simulink model "simpleTVCRocketModel"  (R2021b)
settings: Solver=VariableStepAuto  StartTime=0.0  StopTime=10  RelTol=1e-3
PostLoadFcn:
  | VSS_MODE = 0;
model workspace (MAT data in the model file):
  op_trim6 = opcond.OperatingReport
  op_trim6.Outputs_ = opcond.OutputReport
  op_trim6.Outputs_.yspec_ = 0
  op_trim6.Outputs_.Block_ = 'simpleTVCRocketModel/Theta'
  op_trim6.Outputs_.PortWidth_ = 1
  op_trim6.Outputs_.PortNumber_ = NaN
  op_trim6.Outputs_.Known_ = 0
  op_trim6.Outputs_.Min_ = -Inf
  op_trim6.Outputs_.Max_ = Inf
  op_trim6.TerminationString_ = 'Operating point specifications were successfully met.'
  op_trim6.OptimizationOutput_.iterations = 1
  op_trim6.OptimizationOutput_.funcCount = 9
  op_trim6.OptimizationOutput_.lssteplength = 1
  op_trim6.OptimizationOutput_.stepsize = 0
  op_trim6.OptimizationOutput_.algorithm = 'active-set'
  op_trim6.OptimizationOutput_.firstorderopt = 0
  op_trim6.OptimizationOutput_.constrviolation = 0
  op_trim6.OptimizationOutput_.message = '
    | Local minimum found that satisfies the constraints.
    | 
    | Optimization completed because the objective function is non-decreasing in 
    | feasible directions, to within the value of the optimality tolerance,
    | and constraints are satisfied to within the  value of the constraint tolerance.
    | 
    | <stopping criteria details>
    | 
    | Optimization completed: The first-order optimality measure, 0.000000e+00, is less
    | than options.OptimalityTolerance = 1.000000e-06, and the maximum constraint violation,
    | 0.000000e+00,is less than options.ConstraintTolerance = 1.000000e-06.
    | 
    | '
  op_trim6.OptimizationOutput_.bestfeasible.x = [0; 0; 0; 0; 0; 0; 0; 0]
  op_trim6.OptimizationOutput_.bestfeasible.fval = 0
  op_trim6.OptimizationOutput_.bestfeasible.constrviolation = 0
  op_trim6.OptimizationOutput_.bestfeasible.firstorderopt = 0
  op_trim6.OptimizationOutput_.progress = {'<font face="monospaced"; size=3>', 'Optimizing to solve for all desired dx/dt=0, x(k+1)-x(k)=0, and y=ydes.', ' ', '(Maximum Error)  Block', ' ---------------------------------------------------------', '(0.00000e+00) There are no errors in the operating point search constraints.', '(0.00000e+00) There are no errors in the operating point search constraints.', ' ', 'Operating point specifications were successfully met.'}
  op_trim6.Model_ = 'simpleTVCRocketModel'
  op_trim6.States_(1) = opcond.StateReport
  op_trim6.States_(1).dx_ = [0; 0]
  op_trim6.States_(1).Nx_ = 2
  op_trim6.States_(1).Block_ = 'simpleTVCRocketModel/RocketModel/ASB Rocket Model/Rocket Model/Position'
  op_trim6.States_(1).x_ = [0; 0]
  op_trim6.States_(1).SteadyState_ = [0; 0]
  op_trim6.States_(1).dxMin_ = [-Inf; -Inf]
  op_trim6.States_(1).dxMax_ = [Inf; Inf]
  op_trim6.States_(1).Known_ = [0; 0]
  op_trim6.States_(1).Min_ = [-Inf; -Inf]
  op_trim6.States_(1).Max_ = [Inf; Inf]
  op_trim6.States_(2) = opcond.StateReport
  op_trim6.States_(2).Nx_ = 1
  op_trim6.States_(2).Block_ = 'simpleTVCRocketModel/RocketModel/ASB Rocket Model/Rocket Model/Theta'
  op_trim6.States_(2).SteadyState_ = 1
  op_trim6.States_(2).dxMin_ = -Inf
  op_trim6.States_(2).dxMax_ = Inf
  op_trim6.States_(2).Known_ = 1
  op_trim6.States_(2).Min_ = -Inf
  op_trim6.States_(2).Max_ = Inf
  op_trim6.States_(3) = opcond.StateReport
  op_trim6.States_(3).dx_ = [0; -6.85666666667]
  op_trim6.States_(3).Nx_ = 2
  op_trim6.States_(3).Block_ = 'simpleTVCRocketModel/RocketModel/ASB Rocket Model/Rocket Model/U,w'
  op_trim6.States_(3).x_ = [0; 0]
  op_trim6.States_(3).SteadyState_ = [0; 0]
  op_trim6.States_(3).dxMin_ = [-Inf; -Inf]
  op_trim6.States_(3).dxMax_ = [Inf; Inf]
  op_trim6.States_(3).Known_ = [0; 0]
  op_trim6.States_(3).Min_ = [-Inf; -Inf]
  op_trim6.States_(3).Max_ = [Inf; Inf]
  op_trim6.States_(4) = opcond.StateReport
  op_trim6.States_(4).dx_ = 0
  op_trim6.States_(4).Nx_ = 1
  op_trim6.States_(4).Block_ = 'simpleTVCRocketModel/RocketModel/ASB Rocket Model/Rocket Model/q'
  op_trim6.States_(4).SteadyState_ = 0
  op_trim6.States_(4).dxMin_ = -Inf
  op_trim6.States_(4).dxMax_ = Inf
  op_trim6.States_(4).Known_ = 0
  op_trim6.States_(4).Min_ = -Inf
  op_trim6.States_(4).Max_ = Inf
  op_trim6.States_(5) = opcond.StateReport
  op_trim6.States_(5).Nx_ = 1
  op_trim6.States_(5).Block_ = 'simpleTVCRocketModel/Controller/PID Controller/Filter/Cont. Filter/Filter'
  op_trim6.States_(5).SteadyState_ = 0
  op_trim6.States_(5).dxMin_ = -Inf
  op_trim6.States_(5).dxMax_ = Inf
  op_trim6.States_(5).Known_ = 0
  op_trim6.States_(5).Min_ = -Inf
  op_trim6.States_(5).Max_ = Inf
  op_trim6.States_(6) = opcond.StateReport
  op_trim6.States_(6).Nx_ = 1
  op_trim6.States_(6).Block_ = 'simpleTVCRocketModel/Controller/PID Controller/Integrator/Continuous/Integrator'
  op_trim6.States_(6).SteadyState_ = 0
  op_trim6.States_(6).dxMin_ = -Inf
  op_trim6.States_(6).dxMax_ = Inf
  op_trim6.States_(6).Known_ = 0
  op_trim6.States_(6).Min_ = -Inf
  op_trim6.States_(6).Max_ = Inf
  op_trim6.Inputs_ = opcond.InputReport
  op_trim6.Inputs_.Block_ = 'simpleTVCRocketModel/u'
  op_trim6.Inputs_.PortWidth_ = 1
  op_trim6.Inputs_.PortDimensions_ = [1 1]
  op_trim6.Inputs_.Known_ = 0
  op_trim6.Inputs_.Min_ = -Inf
  op_trim6.Inputs_.Max_ = Inf
libraries: simulink_extras x2, aerolibadyn x1, aerolibconvert2 x1, aerolibanim x1, slpidlib x1, shared3dof x1, simulink x1
settings Model: Creator=joebarnard  LastModifiedBy=willi
settings SolverCC: AlgebraicLoopSolver=TrustRegion
settings DataIOCC: ExternalInput=getinputstruct(op_trim6)  InitialState=getstatestruct(op_trim6)  LoadExternalInput=on  LoadInitialState=on
settings DebuggingCC: SFMachineParentedDataDiag=warning
settings ExplorerConfigSet: InternalSimMechanicsExplorerSettings="<ExplorerConfiguration><canonicalview>default</canonicalview><AnimationSetting><BasePlaybackSpeed>1.0</BasePlaybackSpeed><PlaybackSpeedFactor>1.0</PlaybackSpeedFactor></AnimationSetting><TilePanel><TileInfo><Tiles Columns=\"2\" Count=\"3\" Rows=\"2\"><Column Weight=\"0.5\"/><Column Weight=\"0.5\"/><Row Weight=\"0.5164\"/><Row Weight=\"0.4836\"/><Tile Height=\"1\" Width=\"2\" X=\"0\" Y=\"0\"/><Tile Height=\"1\" Width=\"1\" X=\"0\" Y=\"1\"/><Tile Height=\"1\" Width=\"1\" X=\"1\" Y=\"1\"/></Tiles></TileInfo><SceneInfo><SceneViewer><BGColor><R>0.60000002384185791</R><G>0.60000002384185791</G><B>0.60000002384185791</B></BGColor><Camera><DoPerspective>on</DoPerspective><Position><X>0.0234785756067064089</X><Y>-5.49998084299828705</Y><Z>1.77140121776666781</Z></Position><Center><X>0.0234785756067064089</X><Y>-4.49998084299828705</Y><Z>1.77140121776666781</Z></Center><Up><X>0</X><Y>0</Y><Z>1</Z></Up><ViewLimDist>1</ViewLimDist><YLim>0.466307658154998583</YLim><XLim>1.57644492475456621</XLim></Camera></SceneViewer><SceneViewer><BGColor><R>0.60000002384185791</R><G>0.60000002384185791</G><B>0.60000002384185791</B></BGColor><Camera><DoPerspective>off</DoPerspective><Position><X>1.24658653086195947e-06</X><Y>70.9082318296519531</Y><Z>0.982810102945052222</Z></Position><Center><X>1.24658653086195947e-06</X><Y>-1.81285147970999816e-06</Y><Z>0.982810102945052222</Z></Center><Up><X>0</X><Y>0</Y><Z>1</Z></Up><ViewLimDist>1</ViewLimDist><YLim>28.7116613418530342</YLim><XLim>51.5</XLim></Camera></SceneViewer><SceneViewer><BGColor><R>0.60000002384185791</R><G>0.60000002384185791</G><B>0.60000002384185791</B></BGColor><Camera><DoPerspective>on</DoPerspective><Position><X>0</X><Y>0</Y><Z>3.5</Z></Position><Center><X>0</X><Y>-2.22044604925031308e-16</Y><Z>2.5</Z></Center><Up><X>1</X><Y>0</Y><Z>0</Z></Up><ViewLimDist>1</ViewLimDist><YLim>0.466307658154998583</YLim><XLim>0.836414309469997397</XLim></Camera></SceneViewer></SceneInfo></TilePanel><MechEditorPanel><Cameras><Camera><Id>Camera1</Id><Value><Name>trackCam</Name><NativeCamera><PositionTrackingFeature>RocketModel.Simscape_Rocket_Model.trackCam.R</PositionTrackingFeature><CenterTrackingFeature>RocketModel.Simscape_Rocket_Model.trackCam.R</CenterTrackingFeature><UpVectorTrackingFeature>RocketModel.Simscape_Rocket_Model.trackCam.R</UpVectorTrackingFeature><CenterTrackingOrigin>off</CenterTrackingOrigin><CenterTrackingDirection>-Y</CenterTrackingDirection><UpVectorTrackingDirection>+X</UpVectorTrackingDirection></NativeCamera></Value></Camera><Camera><Id>Camera2</Id><Value><Name>sideTrack</Name><NativeCamera><PositionTrackingFeature>RocketModel.Simscape_Rocket_Model.Camera1.R</PositionTrackingFeature><CenterTrackingFeature>RocketModel.Simscape_Rocket_Model.Camera1.R</CenterTrackingFeature><UpVectorTrackingFeature>RocketModel.Simscape_Rocket_Model.Camera1.R</UpVectorTrackingFeature><CenterTrackingOrigin>off</CenterTrackingOrigin><CenterTrackingDirection>+X</CenterTrackingDirection><UpVectorTrackingDirection>+Y</UpVectorTrackingDirection></NativeCamera></Value></Camera></Cameras><GfxPanelCameraMap><MapElement CameraMLId=\"Camera2\" GfxPanelIndex=\"0\"/><MapElement CameraMLId=\"Camera1\" GfxPanelIndex=\"2\"/></GfxPanelCameraMap><VideoCreator><PlaybackSpeedRatio>1.0</PlaybackSpeedRatio><FrameRate>30</FrameRate><VideoFormat>Motion JPEG AVI</VideoFormat><FrameSize>auto</FrameSize></VideoCreator></MechEditorPanel></ExplorerConfiguration>"

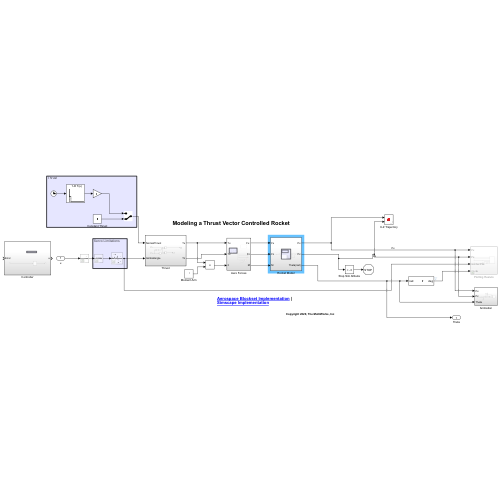
[thumbnail: Simulink's stored preview of the top-level diagram]
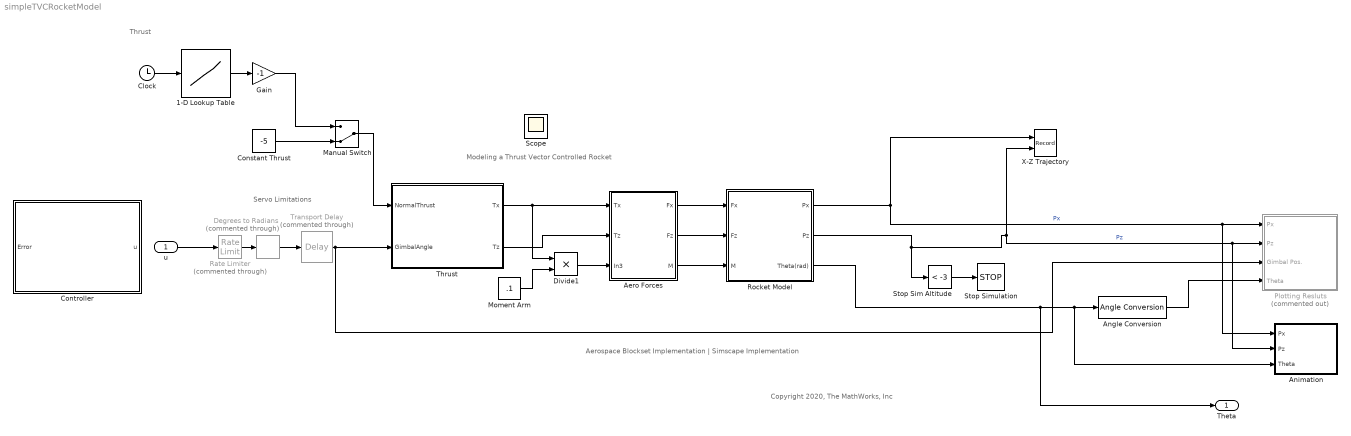
== system simpleTVCRocketModel ==
  note: Servo Limitations
  note: Thrust
  note: Aerospace Blockset Implementation | Simscape Implementation
  note: Modeling a Thrust Vector Controlled Rocket
  note: Copyright 2020, The MathWorks, Inc
  u : Inport
  1-D Lookup Table : Lookup_n-D  NumberOfTableDimensions=1  BreakpointsForDimension1=linspace(0,16.14, 539)  Table=|  InternalRulePriority=Speed  RndMeth=Simplest  InputSameDT=on
      | [0
      | 1.69832354141853
      | 2.47292485439563
      | 4.39373828780983
      | 6.77722955360763
      | 9.10300000000000
      | 11.3977773557748
      | 11.6140807786675
      | 8.98706894846169
      | 6.10838111022478
      | 5.33611774178522
      | 5.01684267037569
      | 5.12969642924522
      | 4.72506262341681
      | 4.73496687053046
      | 4.76034152927576
      | 4.77096696821312
      | 4.76949450279542
      | 4.76619751371507
      | 4.76157438946575
      | 4.75612351854116
      | 4.75034328943497
      | 4.74465776015659
      | 4.73771752958070
      | 4.72923958998768
      | 4.71974568770069
      | 4.70975756904293
      | 4.69979698033756
      | 4.69038566790776
      | 4.68204537807671
      | 4.67529785716758
      | 4.67027632477041
      | 4.66550157069833
      | 4.66080212375550
      | 4.65621865771085
      | 4.65179184633330
      | 4.64756236339179
      | 4.64357088265525
      | 4.63985807789262
      | 4.63646462287282
      | 4.63343119136480
      | 4.63079845713747
      | 4.62860709395979
      | 4.62689777560066
      | 4.62571117582904
      | 4.62508796841385
      | 4.62500000000000
      | 4.62500000000000
      | 4.62500000000000
      | 4.62500000000000
      | 4.62500000000000
      | 4.62500000000000
      | 4.62500000000000
      | 4.62500000000000
      | 4.63106299827402
      | 4.68107635407249
      | 4.75705338209912
      | 4.82903599901373
      | 4.86706612147613
      | 4.86758542991176
      | 4.86569621199534
      | 4.86178755859452
      | 4.85532880808982
      | 4.84578929886178
      | 4.83263836929094
      | 4.81534535775784
      | 4.78894723165560
      | 3.03853849013673
      | 0
      | 0
      | 0
      | 0
      | 0
      | 0
      | 0
      | 0
      | 0
      | 0
      | 0
      | 0
      | 0
      | 0
      | 0
      | 0
      | 0
      | 0
      | 0
      | 0
      | 0
      | 0
      | 0
      | 0
      | 0
      | 0
      | 0
      | 0
      | 0
      | 0
      | 0
      | 0
      | 0
      | 0
      | 0
      | 0
      | 0
      | 0
      | 0
      | 0
      | 0
      | 0
      | 0
      | 0
      | 0
      | 0
      | 0
      | 0
      | 0
      | 0
      | 0
      | 0
      | 0
      | 0
      | 0
      | 0
      | 0
      | 0
      | 0
      | 0
      | 0
      | 0
      | 0
      | 0
      | 0
      | 0
      | 0
      | 0
      | 0
      | 0
      | 0
      | 0
      | 0
      | 0
      | 0
      | 0
      | 0
      | 0
      | 0
      | 0
      | 0
      | 0
      | 0
      | 0
      | 0
      | 0
      | 0
      | 0
      | 0
      | 0
      | 0
      | 0
      | 0
      | 0
      | 0
      | 0
      | 0
      | 0
      | 0
      | 0
      | 0
      | 0
      | 0
      | 0
      | 0
      | 0
      | 0
      | 0
      | 0
      | 0
      | 0
      | 0
      | 0
      | 0
      | 0
      | 0
      | 0
      | 0
      | 0
      | 0
      | 0
      | 0
      | 0
      | 0
      | 0
      | 0
      | 0
      | 0
      | 0
      | 0
      | 0
      | 0
      | 0
      | 0
      | 0
      | 0
      | 0
      | 0
      | 0
      | 0
      | 0
      | 0
      | 0
      | 0
      | 0
      | 0
      | 0
      | 0
      | 0
      | 0
      | 0
      | 0
      | 0
      | 0
      | 0
      | 0
      | 0
      | 0
      | 0
      | 0
      | 0
      | 0
      | 0
      | 0
      | 0
      | 0
      | 0
      | 0
      | 0
      | 0
      | 0
      | 0
      | 0
      | 0
      | 0
      | 0
      | 0
      | 0
      | 0
      | 0
      | 0
      | 0
      | 0
      | 0
      | 0
      | 0
      | 0
      | 0
      | 0
      | 0
      | 0
      | 0
      | 0
      | 0
      | 0
      | 0
      | 0
      | 0
      | 0
      | 0
      | 0
      | 0
      | 0
      | 0
      | 0
      | 0
      | 0
      | 0
      | 0
      | 0
      | 0
      | 0
      | 0
      | 0
      | 0
      | 0
      | 0
      | 0
      | 0
      | 0
      | 0
      | 0
      | 0
      | 0
      | 0
      | 0
      | 0
      | 0
      | 0
      | 0
      | 0
      | 0
      | 0
      | 0
      | 0
      | 0
      | 0
      | 0
      | 0
      | 0
      | 0
      | 0
      | 0
      | 0
      | 0
      | 0
      | 0
      | 0
      | 0
      | 0
      | 0
      | 0
      | 0
      | 0
      | 0
      | 0
      | 0
      | 0
      | 0
      | 0
      | 0
      | 0
      | 0
      | 0
      | 0
      | 0
      | 0
      | 0
      | 0
      | 0
      | 0
      | 0
      | 0
      | 0
      | 0
      | 0
      | 0
      | 0
      | 0
      | 0
      | 0
      | 0
      | 0
      | 0
      | 0
      | 0
      | 0
      | 0
      | 0
      | 0
      | 0
      | 0
      | 0
      | 0
      | 0
      | 0
      | 0
      | 0
      | 0
      | 0
      | 0
      | 0
      | 0
      | 0
      | 0
      | 0
      | 0
      | 0
      | 0
      | 0
      | 0
      | 0
      | 0
      | 0
      | 0
      | 0
      | 0
      | 0
      | 0
      | 0
      | 0
      | 0
      | 0
      | 0
      | 0
      | 0
      | 0
      | 0
      | 0
      | 0
      | 0
      | 0
      | 0
      | 0
      | 0
      | 0
      | 0
      | 0
      | 0
      | 0
      | 0
      | 0
      | 0
      | 0
      | 0
      | 0
      | 0
      | 0
      | 0
      | 0
      | 0
      | 0
      | 0
      | 0
      | 0
      | 0
      | 0
      | 0
      | 0
      | 0
      | 0
      | 0
      | 0
      | 0
      | 0
      | 0
      | 0
      | 0
      | 0
      | 0
      | 0
      | 0
      | 0
      | 0
      | 0
      | 0
      | 0
      | 0
      | 0
      | 0
      | 0
      | 0
      | 0
      | 0
      | 0
      | 0
      | 0
      | 0
      | 0
      | 0
      | 0
      | 0
      | 0
      | 0
      | 0
      | 0
      | 0
      | 0
      | 0
      | 0
      | 0
      | 0
      | 0
      | 0
      | 0
      | 0
      | 0
      | 0
      | 0
      | 0
      | 0
      | 0
      | 0
      | 0
      | 0
      | 0
      | 0
      | 0
      | 0
      | 0
      | 0
      | 0
      | 0
      | 0
      | 0
      | 0
      | 0
      | 0
      | 0
      | 0
      | 0
      | 0
      | 0
      | 0
      | 0
      | 0
      | 0
      | 0
      | 0
      | 0
      | 0
      | 0
      | 0
      | 0
      | 0
      | 0
      | 0
      | 0
      | 0
      | 0
      | 0
      | 0
      | 0
      | 0
      | 0
      | 0
      | 0
      | 0
      | 0
      | 0
      | 0
      | 0
      | 0
      | 0
      | 0
      | 0
      | 0
      | 0
      | 0
      | 0
      | 0]
  Aero Forces : Subsystem
  Angle Conversion : aerolibconvert2/Angle Conversion  IU=rad  OU=deg
  Animation : Subsystem
  Clock : Clock
  Constant Thrust : Constant  Value=-5
  Controller : Subsystem
  Degrees to Radians : simulink_extras/Transformations/Degrees to Radians  Commented=through
  Divide1 : Product  Inputs=**
  Gain : Gain  Gain=-1
  Manual Switch : ManualSwitch  CurrentSetting=0
  "Moment Arm " : Constant  Value=.1
  Plotting Resluts : Subsystem  Commented=on
  Rate Limiter : RateLimiter  Commented=through  RisingSlewLimit=40  FallingSlewLimit=-40  SampleTimeMode=inherited
  Rocket Model : Subsystem
  Stop Sim Altitude : simulink/Logic and Bit Operations/Compare To Constant  relop=<  const=-3  OutDataTypeStr=boolean
  Stop Simulation : Stop
  Thrust : Subsystem
  Transport Delay : TransportDelay  Commented=through  DelayTime=.1
  X-Z Trajectory : Record  FileSettingsInternal="{\"entries\":[{\"content\":{\"excelSettings\":{\"content\":{},\"type\":\"Streamout.ExcelSettings\"}},\"type\":\"Streamout.FileSettingStorage\",\"uuid\":\"8819efe2-75b2-4c39-b171-37ea4a220a1c\"}],\"packageUris\":[\"http://schema.mathworks.com/mf0/streamout_blocks/R2020a\"],\"version\":\"1.0\"}"  Layout=[1 1]  SignalsInternal="{\"entries\":[{\"content\":{\"signals\":[]},\"type\":\"RecordBlkView.InputSignals\",\"uuid\":\"08868f2a-f1b6-4eda-af9c-f928e4978dbd\"}],\"packageUris\":[\"http://schema.mathworks.com/mf0/streamout_blocks/R2020a\"],\"version\":\"1.0\"}"  VisualizationBindings="{\"xyplotplugin\":{\"info\":[{\"series\":[{\"bindingParametersList\":[{\"parameter\":\"X-Axis\",\"signalID\":2843,\"signalName\":\"Px\"},{\"parameter\":\"Y-Axis\",\"signalID\":2847,\"signalName\":\"Pz\"}],\"seriesID\":9305}],\"subplotID\":1}]}}"  CompatibilityTag=XY  st=-1
  Theta : Outport
  Scope : Scope
  wires:
  "Moment Arm "/1 -> Divide1/2
  Thrust/1(Tx) -> Aero Forces/1(Tx), Divide1/1
  Rocket Model/2(Pz) -> Stop Sim Altitude/1, Animation/2(Pz), Plotting Resluts/2(Pz), X-Z Trajectory/2  "Pz"
  Stop Sim Altitude/1 -> Stop Simulation/1
  Rocket Model/1(Px) -> Animation/1(Px), Plotting Resluts/1(Px), X-Z Trajectory/1  "Px"
  1-D Lookup Table/1 -> Gain/1
  Clock/1 -> 1-D Lookup Table/1
  Angle Conversion/1 -> Plotting Resluts/4(Theta)
  Rocket Model/3(Theta(rad)) -> Theta/1, Animation/3(Theta), Angle Conversion/1
  Manual Switch/1 -> Thrust/1(NormalThrust)
  Gain/1 -> Manual Switch/1
  Constant Thrust/1 -> Manual Switch/2
  Aero Forces/1("Fx ") -> Rocket Model/1(Fx)
  Thrust/2(Tz) -> Aero Forces/2(Tz)
  Aero Forces/2(Fz) -> Rocket Model/2(Fz)
  Aero Forces/3(M) -> Rocket Model/3(M)
  Divide1/1 -> Aero Forces/3(In3)
  Transport Delay/1 -> Plotting Resluts/3(Gimbal Pos.), Thrust/2(GimbalAngle)
  Rate Limiter/1 -> Degrees to Radians/1
  Degrees to Radians/1 -> Transport Delay/1
  u/1 -> Rate Limiter/1

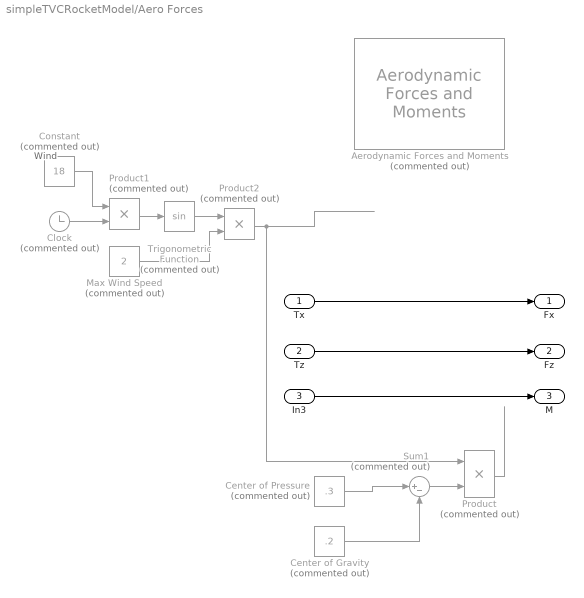
== system simpleTVCRocketModel/Aero Forces ==
  note: Wind
  Tx : Inport
  Tz : Inport  Port=2
  In3 : Inport  Port=3
  "Aerodynamic Forces and Moments " : aerolibadyn/Aerodynamic Forces and Moments   Commented=on  inputAxes=Body  outputForceAxes=Body  outputMomentAxes=Body  S=1  b=1  cbar=1
  Center of Gravity : Constant  Commented=on  Value=.2
  Center of Pressure : Constant  Commented=on  Value=.3
  Clock : Clock  Commented=on
  Constant : Constant  Commented=on  Value=18
  Max Wind Speed : Constant  Commented=on  Value=2
  Product : Product  Commented=on
  Product1 : Product  Commented=on
  Product2 : Product  Commented=on
  Sum1 : Sum  Commented=on  Inputs=|+-
  Trigonometric Function : Trigonometry  Commented=on
  "Fx " : Outport
  Fz : Outport  Port=2
  M : Outport  Port=3
  wires:
  Tz/1 -> Fz/1
  Product1/1 -> Trigonometric Function/1
  Clock/1 -> Product1/2
  Constant/1 -> Product1/1
  Trigonometric Function/1 -> Product2/1
  Tx/1 -> "Fx "/1
  Center of Pressure/1 -> Sum1/1
  Center of Gravity/1 -> Sum1/2
  Sum1/1 -> Product/2
  In3/1 -> M/1
  Product/1 -> ?
  Product2/1 -> Product/1
  Max Wind Speed/1 -> Product2/2

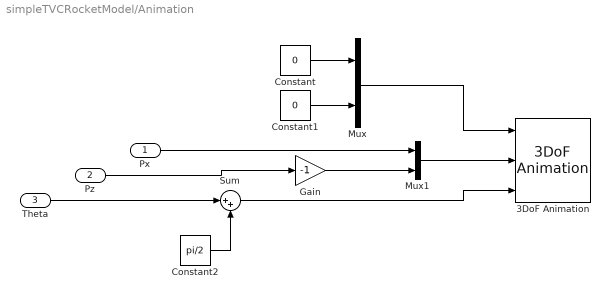
== system simpleTVCRocketModel/Animation ==
  Px : Inport
  Pz : Inport  Port=2
  Theta : Inport  Port=3
  3DoF Animation : aerolibanim/3DoF Animation  u1=[-10 10 -10 10 0 50]  u2=.01  u3=.1  u5=Fixed position  u6=[0 -100 0]  u7=10  u8=on
      settings: SourceProductBaseCode=AE
  Constant : Constant  Value=0
  Constant1 : Constant  Value=0
  Constant2 : Constant  Value=pi/2
  Gain : Gain  Gain=-1
  Mux : Mux  Inputs=2
  Mux1 : Mux  Inputs=2
  Sum : Sum  Inputs=|++
  wires:
  Constant/1 -> Mux/1
  Theta/1 -> Sum/1
  Constant2/1 -> Sum/2
  Mux/1 -> 3DoF Animation/1
  Px/1 -> Mux1/1
  Sum/1 -> 3DoF Animation/3
  Mux1/1 -> 3DoF Animation/2
  Constant1/1 -> Mux/2
  Pz/1 -> Gain/1
  Gain/1 -> Mux1/2

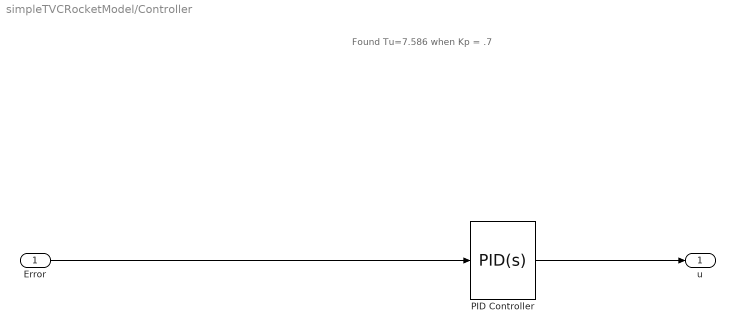
== system simpleTVCRocketModel/Controller ==
  note: Found Tu=7.586 when Kp = .7
  Error : Inport
  PID Controller : slpidlib/PID Controller  Controller=PID  Form=Parallel  TimeDomain=Continuous-time  UseExternalTs=off  SampleTime=-1  IntegratorMethod=Forward Euler  FilterMethod=Forward Euler  ControllerParametersSource=internal  P=1  I=0  D=0  UseFilter=on  N=100  TunerSelectOption=Transfer Function Based (PID Tuner App)  InitialConditionSource=internal  InitialConditionForIntegrator=0  InitialConditionForFilter=0  DifferentiatorICPrevScaledInput=0  ExternalReset=none  TrackingMode=off  Kt=1  LimitOutput=on  SatLimitsSource=internal  UpperSaturationLimit=5  LowerSaturationLimit=-5  LinearizeAsGain=off  AntiWindupMode=none  Kb=1  POutMin=[]  POutMax=[]  IOutMin=[]  IOutMax=[]  DOutMin=[]  DOutMax=[]  NOutMin=[]  NOutMax=[]  SumOutMin=[]  SumOutMax=[]  SaturationOutMin=[]  SaturationOutMax=[]  PParamMin=[]  PParamMax=[]  IParamMin=[]  IParamMax=[]  DParamMin=[]  DParamMax=[]  NParamMin=[]  NParamMax=[]  KbParamMin=[]  KbParamMax=[]  KtParamMin=[]  KtParamMax=[]  KbOutMin=[]  KbOutMax=[]  KtOutMin=[]  KtOutMax=[]  IntegratorOutMin=[]  IntegratorOutMax=[]  FilterOutMin=[]  FilterOutMax=[]  SumI1OutMin=[]  SumI1OutMax=[]  SumI2OutMin=[]  SumI2OutMax=[]  SumI3OutMin=[]  SumI3OutMax=[]  SumI4OutMin=[]  SumI4OutMax=[]  SumDOutMin=[]  SumDOutMax=[]  DifferentiatorOutMin=[]  DifferentiatorOutMax=[]  FilterDiffOutCoefMin=[]  FilterDiffOutCoefMax=[]  ReciprocalOutMin=[]  ReciprocalOutMax=[]  SumDenOutMin=[]  SumDenOutMax=[]  SumNumOutMin=[]  SumNumOutMax=[]  DivideOutMin=[]  DivideOutMax=[]  UdiffTsProdOutMin=[]  UdiffTsProdOutMax=[]  NTsProdOutMin=[]  NTsProdOutMax=[]  UintegralTsProdOutMin=[]  UintegralTsProdOutMax=[]  UngainTsProdOutMin=[]  UngainTsProdOutMax=[]  IntegratorContinuousStateAttributes=''  IntegratorStateMustResolveToSignalObject=off  IntegratorRTWStateStorageClass=Auto  FilterContinuousStateAttributes=''  FilterStateMustResolveToSignalObject=off  FilterRTWStateStorageClass=Auto  ParallelPVariant=InternalParameters  IdealPVariant=Disabled  IVariant=InternalParameters  DVariant=InternalParameters  IntegratorVariant=Continuous  SatVariant=Enabled  AWVariant=Passthrough  PCopyVariant=Disabled  TRVariant=Disabled  FdbkBlocksVariant=Forward  IdealPFdbkVariant=Disabled  SatFdbkVariant=Disabled  DerivativeFilterVariant=ContFilter  NVariant=InternalParameters  NCopyVariant=Disabled  FilterICVariant=InternalICsFilter  IntegratorICVariant=InternalICs  ExternalResetVariant=Disabled  TRSumVariant=Passthrough  SumFdbkVariant=Disabled  SumVariant=Sum_PID  TsampFilterVariant=InternalTs  TsampNgainVariant=Passthrough  TsampIntegralVariant=Passthrough  ExternalSaturationOutDataTypeStr=Inherit: Same as second input
  u : Outport
  wires:
  Error/1 -> PID Controller/1
  PID Controller/1 -> u/1

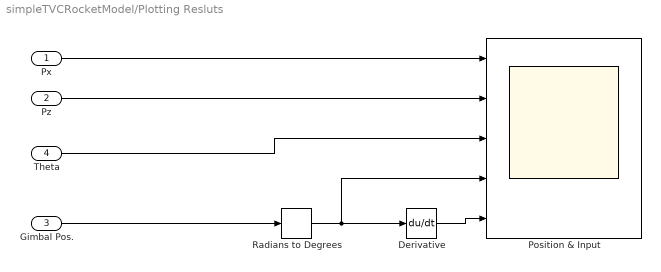
== system simpleTVCRocketModel/Plotting Resluts ==
  Px : Inport
  Pz : Inport  Port=2
  Gimbal Pos. : Inport  Port=3
  Theta : Inport  Port=4
  Derivative : Derivative
  Position & Input : Scope  NumInputPorts=5
  Radians to Degrees : simulink_extras/Transformations/Radians to Degrees
      link override Gain: Gain=57.2957795130823
  wires:
  Px/1 -> Position & Input/1
  Derivative/1 -> Position & Input/5
  Pz/1 -> Position & Input/2
  Radians to Degrees/1 -> Derivative/1, Position & Input/4
  Gimbal Pos./1 -> Radians to Degrees/1
  Theta/1 -> Position & Input/3

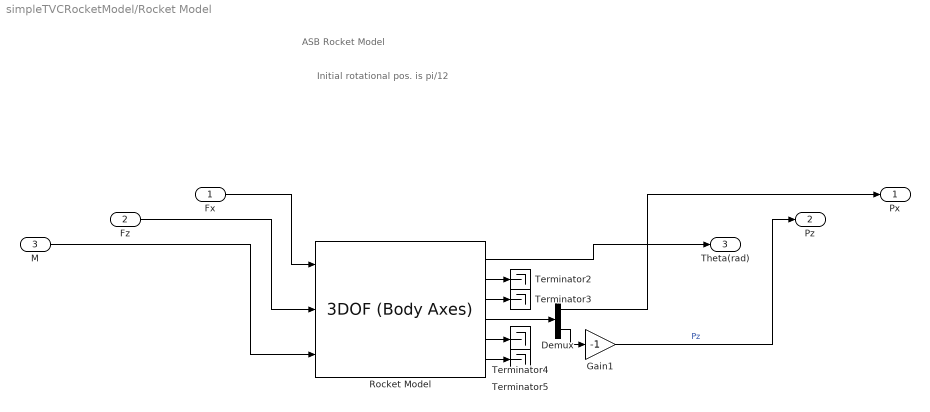
== system simpleTVCRocketModel/Rocket Model ==
  note: Initial rotational pos. is pi/12
  note: ASB Rocket Model
  Fx : Inport
  Fz : Inport  Port=2
  M : Inport  Port=3
  Demux : Demux  Outputs=2
  Gain1 : Gain  Gain=-1
  Rocket Model : shared3dof/3DOF (Body Axes)  units=Metric (MKS)  mtype=Fixed  v_ini=0  theta_ini=Initial_Body_Attitude  alpha_ini=0  pos_ini=[0 0]  q_ini=0  mass=Initial_Mass_of_Rocket  mass_e=0.5  mass_f=3.0  Iyy=.075  Iyy_e=0.5  Iyy_f=3.0  g_in=Internal  g=9.81  vre_flag=on  abi_flag=off  aMode=0  vel_statename=''  theta_statename=''  pos_statename=''  q_statename=''  mass_statename=''
      settings: SourceProductBaseCode=AE,PW,DR,MT,UV,VE
  Terminator{2..5} (4 alike) : Terminator
  Px : Outport
  Pz : Outport  Port=2
  Theta(rad) : Outport  Port=3
  wires:
  Fx/1 -> Rocket Model/1
  Rocket Model/1 -> Theta(rad)/1
  Rocket Model/5 -> Terminator4/1
  Demux/1 -> Px/1
  M/1 -> Rocket Model/3
  Gain1/1 -> Pz/1  "Pz"
  Fz/1 -> Rocket Model/2
  Demux/2 -> Gain1/1
  Rocket Model/2 -> Terminator2/1
  Rocket Model/6 -> Terminator5/1
  Rocket Model/4 -> Demux/1
  Rocket Model/3 -> Terminator3/1

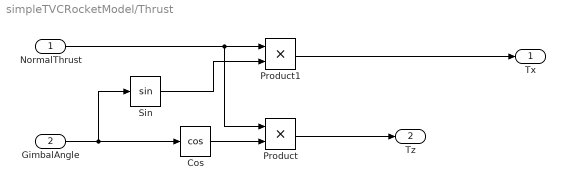
== system simpleTVCRocketModel/Thrust ==
  NormalThrust : Inport
  GimbalAngle : Inport  Port=2
  Cos : Trigonometry  Operator=cos
  Product : Product  RndMeth=Zero
  Product1 : Product  RndMeth=Zero
  Sin : Trigonometry
  Tx : Outport
  Tz : Outport  Port=2
  wires:
  GimbalAngle/1 -> Cos/1, Sin/1
  Product/1 -> Tz/1
  Cos/1 -> Product/2
  NormalThrust/1 -> Product/1, Product1/1
  Sin/1 -> Product1/2
  Product1/1 -> Tx/1
